simulink model "regulatorsimexp"  (Simulink 5.0)
settings: Solver=ode45  StartTime=0.0  StopTime=Tstop  RelTol=1e-3
values from neighbouring files (symbols this model uses):
  Cexp = expcon(Cimp,range)    [doubleintexp.m]    (also in example2.m = expcon(Cimp,range,options); mexexample1.m; regsiso.m; regulator.m)
  x10 = 2    [regulator.m]
  x20 = 3    [regulator.m]
libraries: hyblib x1, simulink x1
settings Model: LastModifiedBy=Alberto Bemporad  OptimizeBlockIOStorage=off

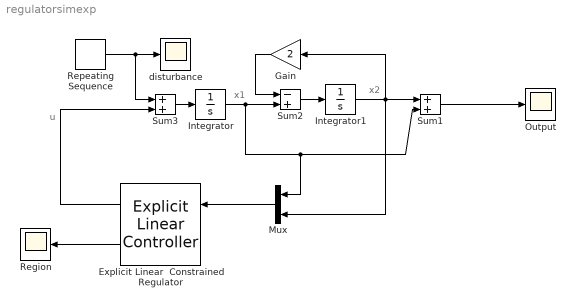
== system regulatorsimexp ==
  note: x2
  note: x1
  note: u
  Explicit Linear  Constrained Regulator : hyblib/Explicit Linear Controller  Orientation=left  C=Cexp  xhat0=[]  u1=[]  compile=on
  Gain : Gain  Orientation=left  Gain=2  SaturateOnIntegerOverflow=on
  Integrator : Integrator  InitialCondition=x10
  Integrator1 : Integrator  InitialCondition=x20
  Mux : Mux  Orientation=left  Inputs=2
  Output : Scope
      settings: TimeRange=30  YMin=-2  YMax=8
  Region : Scope
      settings: TimeRange=30  YMin=1  YMax=4
  Repeating Sequence : simulink/Sources/Repeating Sequence  rep_seq_t=[0 .1 10]  rep_seq_y=[30 0 0]
  Sum1 : Sum  SaturateOnIntegerOverflow=on
  Sum2 : Sum  Inputs=-+  SaturateOnIntegerOverflow=on
  Sum3 : Sum  SaturateOnIntegerOverflow=on
  disturbance : Scope
      settings: TimeRange=30  YMin=0  YMax=30  SaveName=ScopeData2
  wires:
  Integrator1/1 -> Gain/1, Sum1/1, Mux/2
  Sum2/1 -> Integrator1/1
  Integrator/1 -> Sum2/2, Sum1/2, Mux/1
  Gain/1 -> Sum2/1
  Sum1/1 -> Output/1
  Explicit Linear  Constrained Regulator/2 -> Region/1
  Sum3/1 -> Integrator/1
  Repeating Sequence/1 -> Sum3/1, disturbance/1
  Explicit Linear  Constrained Regulator/1 -> Sum3/2
  Mux/1 -> Explicit Linear  Constrained Regulator/1
